simulink model "Cascade_realization"  (R2020b)
settings: Solver=VariableStepAuto  StartTime=0.0  StopTime=10.0  RelTol=1e-3
settings Model: Creator=saadh  LastModifiedBy=saadh
settings DataIOCC: SaveOutput=off  SaveTime=off

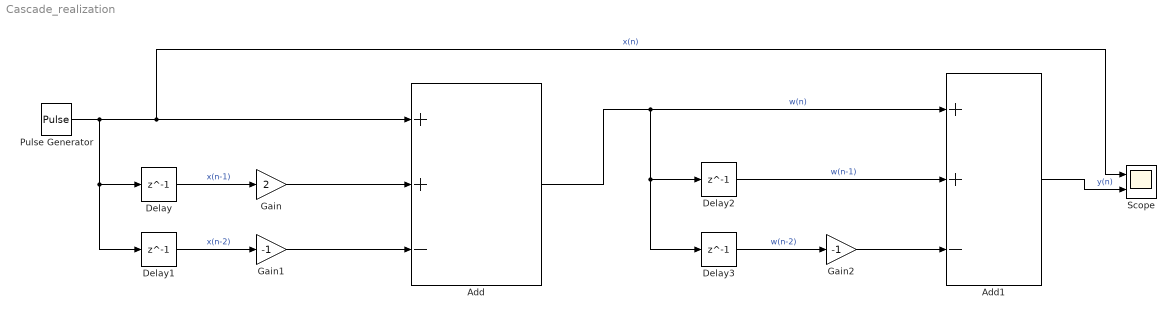
== system Cascade_realization ==
  Add : Sum  Inputs=++-
  Add1 : Sum  Inputs=++-
  Delay{,1..3} (4 alike) : Delay  DelayLength=1
  Gain : Gain  Gain=2
  Gain1 : Gain  Gain=-1
  Gain2 : Gain  Gain=-1
  Pulse Generator : DiscretePulseGenerator  PulseType=Time based  Period=1  PulseWidth=5
  Scope : Scope  NumInputPorts=2
  wires:
  Add1/1 -> Scope/2  "y(n)"
  Delay/1 -> Gain/1  "x(n-1)"
  Delay2/1 -> Add1/2  "w(n-1)"
  Pulse Generator/1 -> Add/1, Scope/1, Delay/1, Delay1/1  "x(n)"
  Add/1 -> Add1/1, Delay2/1, Delay3/1  "w(n)"
  Gain/1 -> Add/2
  Delay1/1 -> Gain1/1  "x(n-2)"
  Gain2/1 -> Add1/3
  Gain1/1 -> Add/3
  Delay3/1 -> Gain2/1  "w(n-2)"
